simulink model "linctrl_k"  (R2021a)
settings: Solver=VariableStepAuto  StartTime=0.0  StopTime=tf  FixedStep=1/365  RelTol=1e-3
values from neighbouring files (symbols this model uses):
  apply_noise = 1    [fbl.m]
  noise_a = -20e-7    (= -2e-06)    [main.m]
  noise_b = -50e-7    (= -5e-06)    [main.m]
  r = 0    [main.m]
  Ts = 0.02    [main.m]
  x0 = [950; 550; 6e-4]    [main.m]
  x10 = 1000    [main.m]
  x20 = 550    [main.m]
undefined symbols (not defined in the file or in its folder): k_p
libraries: simulink x1
settings Model: Creator=micma  LastModifiedBy=micma

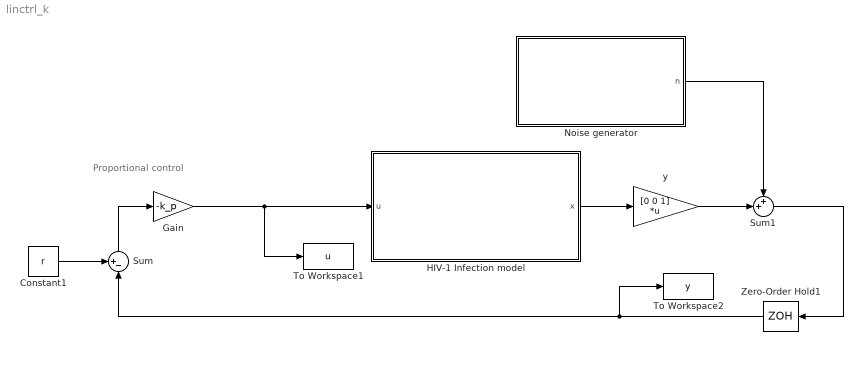
== system linctrl_k ==
  note: Proportional control
  Constant1 : Constant  Value=r
  Gain : Gain  Gain=-k_p
  HIV-1 Infection model : Subsystem
  Noise generator : Subsystem
  Sum : Sum  Inputs=+-|
  Sum1 : Sum  Inputs=++|
  To Workspace1 : ToWorkspace  VariableName=u  SaveFormat=Timeseries  SampleTime=-1
  To Workspace2 : ToWorkspace  VariableName=y  SaveFormat=Timeseries  SampleTime=-1
  Zero-Order Hold1 : ZeroOrderHold  SampleTime=Ts
  y : Gain  Gain=[0 0 1]  Multiplication=Matrix(K*u)
  wires:
  Sum/1 -> Gain/1
  Constant1/1 -> Sum/1
  Gain/1 -> HIV-1 Infection model/1(u), To Workspace1/1
  HIV-1 Infection model/1(x) -> y/1
  Zero-Order Hold1/1 -> Sum/2, To Workspace2/1
  y/1 -> Sum1/2
  Noise generator/1(n) -> Sum1/1
  Sum1/1 -> Zero-Order Hold1/1

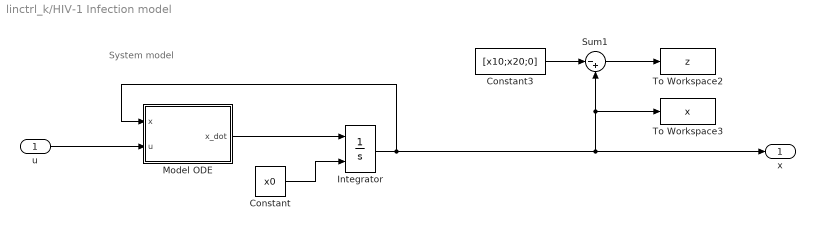
== system linctrl_k/HIV-1 Infection model ==
  note: System model
  u : Inport
  Constant : Constant  Value=x0
  Constant3 : Constant  Value=[x10;x20;0]
  Integrator : Integrator  InitialConditionSource=external
  Model ODE : MATLAB Function  TreatAsAtomicUnit=on
  Sum1 : Sum  Inputs=|-+
  To Workspace2 : ToWorkspace  VariableName=z  SaveFormat=Timeseries  SampleTime=-1
  To Workspace3 : ToWorkspace  VariableName=x  SaveFormat=Timeseries  SampleTime=-1
  x : Outport
  wires:
  Model ODE/1(x_dot) -> Integrator/1
  Constant/1 -> Integrator/2
  Constant3/1 -> Sum1/1
  Sum1/1 -> To Workspace2/1
  Integrator/1 -> To Workspace3/1, Sum1/2, x/1, Model ODE/1(x)
  u/1 -> Model ODE/2(u)

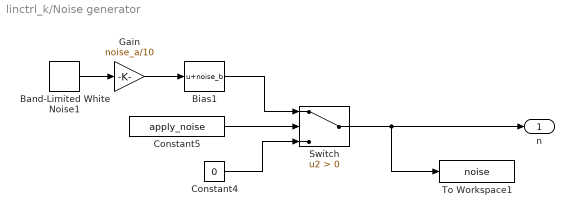
== system linctrl_k/Noise generator ==
  Band-Limited White Noise1 : simulink/Sources/Band-Limited White Noise  Cov=[.1]  Ts=Ts*0.1  seed=[23341]
  Bias1 : Bias  Bias=noise_b
  Constant4 : Constant  Value=0
  Constant5 : Constant  Value=apply_noise
  Gain : Gain  Gain=noise_a/10
  Switch : Switch  Criteria=u2 > Threshold
  To Workspace1 : ToWorkspace  VariableName=noise  SaveFormat=Timeseries  SampleTime=-1
  n : Outport
  wires:
  Constant5/1 -> Switch/2
  Constant4/1 -> Switch/3
  Switch/1 -> n/1, To Workspace1/1
  Bias1/1 -> Switch/1
  Band-Limited White Noise1/1 -> Gain/1
  Gain/1 -> Bias1/1

== matlab function linctrl_k/HIV-1 Infection model/Model ODE ==
  data: x input; u input; x_dot output; params parameter
function x_dot = ode(x, u, params)
x_dot = modelODE(x, u, params);
end
